simulink model "lqr_outer_test"  (R2017a)
settings: Solver=ode4  StartTime=0.0  StopTime=5  FixedStep=Ts  RelTol=1e-3  EnableMultiTasking=on
values from neighbouring files (symbols this model uses):
  Ac = [0 0 0  1 0 0   0  0  0  0 ... (first row only)    [lqr_outer_synthesis.m]
  Bc = [zeros(3,3) ... (first row only)    [lqr_outer_synthesis.m]
  Cc = [eye(3) zeros(3,7)]    [lqr_outer_synthesis.m]
  Ki_lqr = [0  0  8.66025403784; 0  -0.1  0; 0.1  0  0]    [K_lqr.mat]    (also in lqr_outer_synthesis.m = -K(:,11:end))
  Kx_lqr = [0 0 0.263619393691 0 -0.257300038922 0 13.6588017709 0 0 0 0 0.247475923649 ... (30 elements, 3x10)]    [K_lqr.mat]    (also in lqr_outer_synthesis.m = K(:,1:10))
undefined symbols (not defined in the file or in its folder): B_inner_inv, gra, KT, mass
settings Model: Creator=dtnguyen  LastModifiedBy=ducnguyen
settings DataIOCC: LimitDataPoints=on  SaveFormat=Array
settings OptimizationCC: DefaultParameterBehavior=Inlined  UseFloatMulNetSlope=on  InlineInvariantSignals=on  EfficientFloat2IntCast=on  LifeSpan=inf
settings DebuggingCC: SFUnexpectedBacktrackingDiag=warning  SFNoUnconditionalDefaultTransitionDiag=warning  SFExecutionAtInitializationDiag=none
settings HardwareCC: ProdBitPerPointer=32  ProdBitPerSizeT=32  ProdBitPerPtrDiffT=32  ProdLargestAtomicFloat=None  ProdIntDivRoundTo=Undefined  ProdEndianess=Unspecified  ProdWordSize=32  ProdHWDeviceType=32-bit Generic
settings ModelReferenceCC: PropagateSignalLabelsOutOfModel=off
settings RTWCC: GenerateReport=on  Toolchain=Catkin  BuildConfiguration=Faster Runs  LaunchReport=on  TargetLang=C++  CheckMdlBeforeBuild=Warning
settings GRTTargetCC: TargetLangStandard=C++03 (ISO)  GeneratePreprocessorConditionals=Disable all  MatFileLogging=off  MultiInstanceERTCode=on  CodeInterfacePackaging=C++ class  SupportNonFinite=off
settings ConfigComp: CovMetricSettings=dw  CovHtmlReporting=on  CovSaveCumulativeToWorkspaceVar=on  CovSaveSingleToWorkspaceVar=on  CovExternalEMLEnable=off

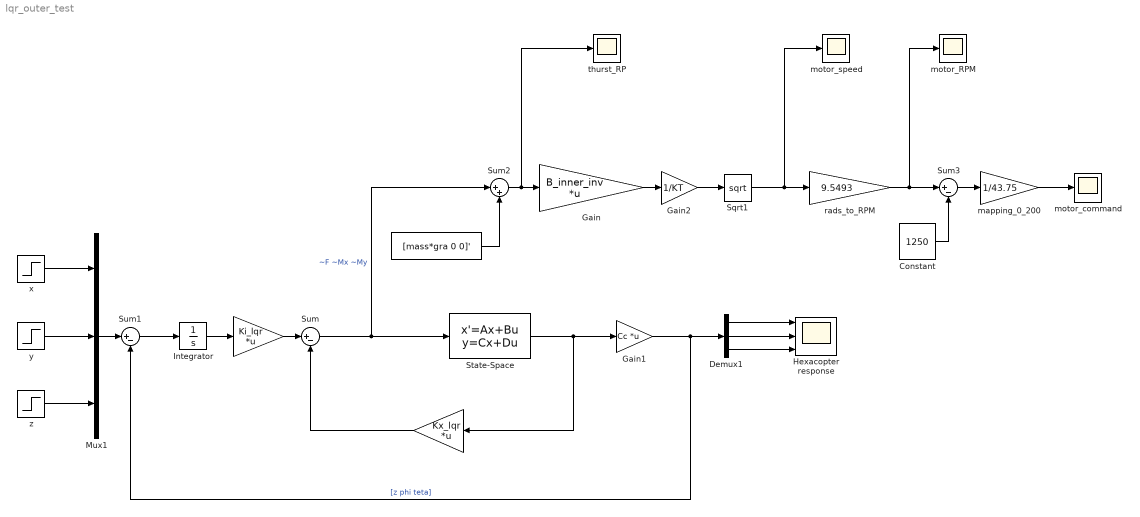
== system lqr_outer_test ==
  " " : Gain  Gain=Ki_lqr  Multiplication=Matrix(K*u)
  "              " : Constant  Value=[mass*gra 0 0]'
  "                   " : Gain  Gain=Kx_lqr  Multiplication=Matrix(K*u)
  Constant : Constant  Value=1250  VectorParams1D=off  SampleTime=-1
  Demux1 : Demux  Outputs=3
  Gain : Gain  Gain=B_inner_inv  Multiplication=Matrix(K*u)
  Gain1 : Gain  Gain=Cc  Multiplication=Matrix(K*u)
  Gain2 : Gain  Gain=1/KT
  Hexacopter response : Scope  NumInputPorts=3
  Integrator : Integrator  InitialCondition=[0 0 0]
  Mux1 : Mux  Inputs=3
  Sqrt1 : Sqrt  SaturateOnIntegerOverflow=on
  State-Space : StateSpace  A=Ac  B=Bc  C=eye(10)  D=zeros(10,3)  X0=0
  Sum : Sum  Inputs=|+-
  Sum1 : Sum  Inputs=|+-
  Sum2 : Sum  Inputs=|++
  Sum3 : Sum  Inputs=|+-
  mapping_0_200 : Gain  Gain=1/43.75
  motor_RPM : Scope
  motor_command : Scope
  motor_speed : Scope
  rads_to_RPM : Gain  Gain=9.5493
  thurst_RP : Scope
  x : Step  Time=0  After=0  SampleTime=0
  y : Step  Time=0  After=0  SampleTime=0
  z : Step  Time=0  After=0.5  SampleTime=0
  wires:
  Sum/1 -> Sum2/1, State-Space/1  "~F ~Mx ~My"
  "                   "/1 -> Sum/2
  Integrator/1 -> " "/1
  " "/1 -> Sum/1
  Mux1/1 -> Sum1/1
  Demux1/2 -> Hexacopter response/2
  Demux1/1 -> Hexacopter response/1
  Demux1/3 -> Hexacopter response/3
  z/1 -> Mux1/3
  x/1 -> Mux1/1
  y/1 -> Mux1/2
  Sum1/1 -> Integrator/1
  State-Space/1 -> Gain1/1, "                   "/1
  Gain1/1 -> Sum1/2, Demux1/1  "[z phi teta]"
  "              "/1 -> Sum2/2
  Sum2/1 -> thurst_RP/1, Gain/1
  Gain/1 -> Gain2/1
  Gain2/1 -> Sqrt1/1
  Sqrt1/1 -> rads_to_RPM/1, motor_speed/1
  rads_to_RPM/1 -> Sum3/1, motor_RPM/1
  mapping_0_200/1 -> motor_command/1
  Constant/1 -> Sum3/2
  Sum3/1 -> mapping_0_200/1
